simulink model "Longitudinal_Vehicle_Control"  (R2021a)
settings: Solver=VariableStepAuto  StartTime=0.0  StopTime=20  RelTol=1e-3
settings Model: Creator=AK  LastModifiedBy=AK

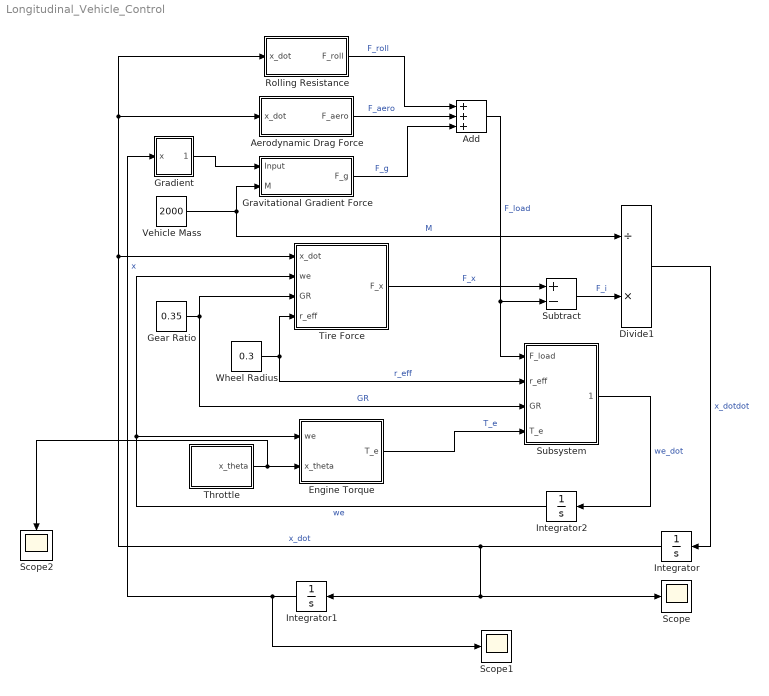
== system Longitudinal_Vehicle_Control ==
  Add : Sum  Inputs=+++
  Aerodynamic Drag Force : Subsystem
  Divide1 : Product  Inputs=/*
  Engine Torque : Subsystem
  Gear Ratio : Constant  Value=0.35
  Gradient : Subsystem
  Gravitational Gradient Force : Subsystem
  Integrator : Integrator  InitialCondition=5
  Integrator1 : Integrator
  Integrator2 : Integrator  InitialCondition=100
  Rolling Resistance : Subsystem
  Scope : Scope
  Scope1 : Scope
  Scope2 : Scope
  Subsystem : Subsystem
  Subtract : Sum  Inputs=+-
  Throttle : Subsystem
  Tire Force : Subsystem
  Vehicle Mass : Constant  Value=2000
  Wheel Radius : Constant  Value=0.3
  wires:
  Vehicle Mass/1 -> Divide1/1, Gravitational Gradient Force/2(M)  "M"
  Divide1/1 -> Integrator/1  "x_dotdot"
  Integrator/1 -> Scope/1, Integrator1/1, Tire Force/1(x_dot), Aerodynamic Drag Force/1(x_dot), Rolling Resistance/1(x_dot)  "x_dot"
  Add/1 -> Subtract/2, Subsystem/1(F_load)  "F_load"
  Gear Ratio/1 -> Subsystem/3(GR), Tire Force/3(GR)  "GR"
  Wheel Radius/1 -> Subsystem/2(r_eff), Tire Force/4(r_eff)  "r_eff"
  Integrator2/1 -> Tire Force/2(we), Engine Torque/1(we)  "we"
  Subtract/1 -> Divide1/2  "F_i"
  Aerodynamic Drag Force/1(F_aero) -> Add/2  "F_aero"
  Rolling Resistance/1(F_roll) -> Add/1  "F_roll"
  Gravitational Gradient Force/1(F_g) -> Add/3  "F_g"
  Tire Force/1(F_x) -> Subtract/1  "F_x"
  Engine Torque/1(T_e) -> Subsystem/4(T_e)  "T_e"
  Subsystem/1(we_dot) -> Integrator2/1  "we_dot"
  Integrator1/1 -> Scope1/1, Gradient/1(x)  "x"
  Gradient/1(alpha) -> Gravitational Gradient Force/1(Input)
  Throttle/1(x_theta) -> Scope2/1, Engine Torque/2(x_theta)

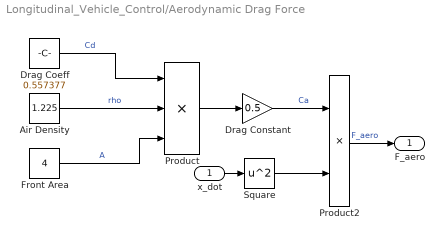
== system Longitudinal_Vehicle_Control/Aerodynamic Drag Force ==
  x_dot : Inport
  Air Density : Constant  Value=1.225
  Drag Coeff : Constant  Value=0.557377
  Drag Constant : Gain  Gain=0.5
  Front Area : Constant  Value=4
  Product : Product  Inputs=3
  Product2 : Product
  Square : Math  Operator=square  SaturateOnIntegerOverflow=on
  F_aero : Outport
  wires:
  Drag Constant/1 -> Product2/1  "Ca"
  Product/1 -> Drag Constant/1
  Air Density/1 -> Product/2  "rho"
  Drag Coeff/1 -> Product/1  "Cd"
  Square/1 -> Product2/2
  Product2/1 -> F_aero/1  "F_aero"
  Front Area/1 -> Product/3  "A"
  x_dot/1 -> Square/1

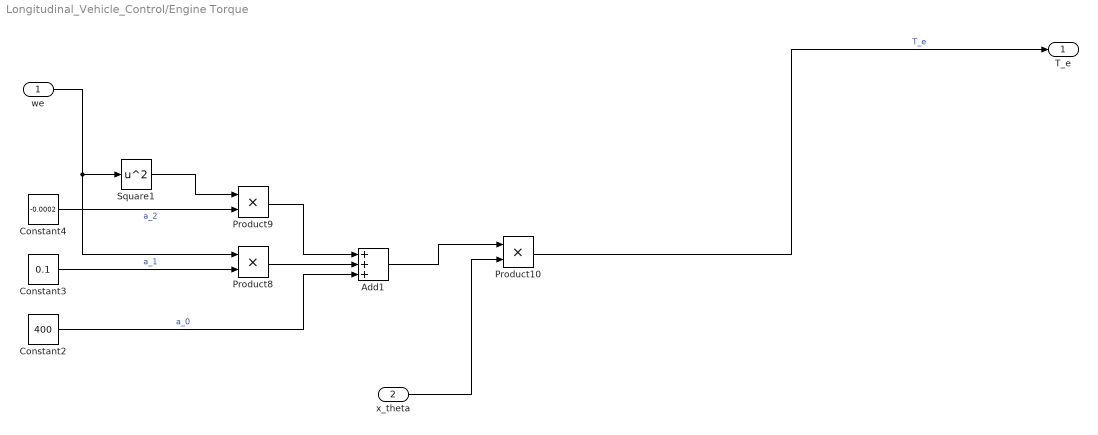
== system Longitudinal_Vehicle_Control/Engine Torque ==
  we : Inport
  x_theta : Inport  Port=2
  Add1 : Sum  Inputs=+++
  Constant2 : Constant  Value=400
  Constant3 : Constant  Value=0.1
  Constant4 : Constant  Value=-0.0002
  Product10 : Product
  Product8 : Product
  Product9 : Product
  Square1 : Math  Operator=square  SaturateOnIntegerOverflow=on
  T_e : Outport
  wires:
  Square1/1 -> Product9/1
  Add1/1 -> Product10/1
  Constant4/1 -> Product9/2  "a_2"
  we/1 -> Product8/1, Square1/1
  Product9/1 -> Add1/1
  Constant3/1 -> Product8/2  "a_1"
  Product8/1 -> Add1/2
  Constant2/1 -> Add1/3  "a_0"
  Product10/1 -> T_e/1  "T_e"
  x_theta/1 -> Product10/2

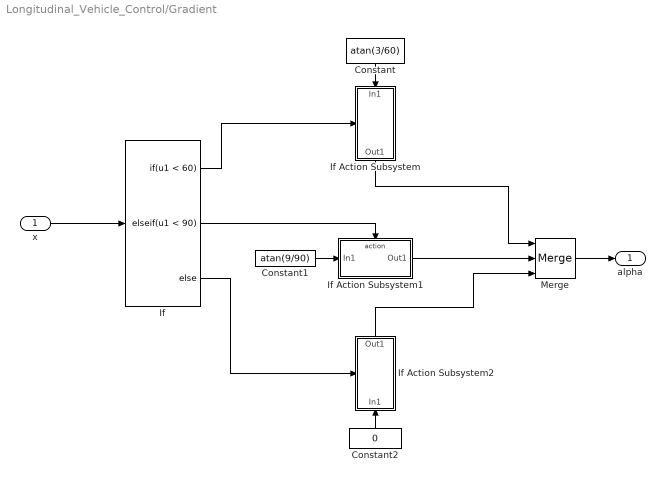
== system Longitudinal_Vehicle_Control/Gradient ==
  x : Inport
  Constant : Constant  Value=atan(3/60)
  Constant1 : Constant  Value=atan(9/90)
  Constant2 : Constant  Value=0
  If : If  IfExpression=u1 < 60  ElseIfExpressions=u1 < 90
  If Action Subsystem : Subsystem  TreatAsAtomicUnit=on
  If Action Subsystem1 : Subsystem  TreatAsAtomicUnit=on
  If Action Subsystem2 : Subsystem  TreatAsAtomicUnit=on
  Merge : Merge  Inputs=3
  alpha : Outport
  wires:
  x/1 -> If/1
  If/1 -> If Action Subsystem/Action
  Constant/1 -> If Action Subsystem/1(In1)
  Constant1/1 -> If Action Subsystem1/1(In1)
  If/2 -> If Action Subsystem1/Action
  Constant2/1 -> If Action Subsystem2/1(In1)
  If/3 -> If Action Subsystem2/Action
  If Action Subsystem/1(Out1) -> Merge/1
  If Action Subsystem1/1(Out1) -> Merge/2
  If Action Subsystem2/1(Out1) -> Merge/3
  Merge/1 -> alpha/1

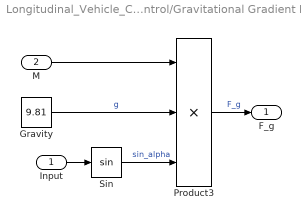
== system Longitudinal_Vehicle_Control/Gravitational Gradient Force ==
  Input : Inport
  M : Inport  Port=2
  Gravity : Constant  Value=9.81
  Product3 : Product  Inputs=3
  Sin : Trigonometry
  F_g : Outport
  wires:
  Sin/1 -> Product3/3  "sin_alpha"
  Gravity/1 -> Product3/2  "g"
  M/1 -> Product3/1
  Product3/1 -> F_g/1  "F_g"
  Input/1 -> Sin/1

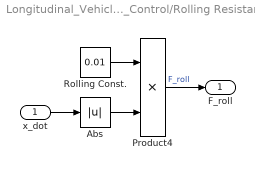
== system Longitudinal_Vehicle_Control/Rolling Resistance ==
  x_dot : Inport
  Abs : Abs
  Product4 : Product
  Rolling Const. : Constant  Value=0.01
  F_roll : Outport
  wires:
  Product4/1 -> F_roll/1  "F_roll"
  Rolling Const./1 -> Product4/1
  Abs/1 -> Product4/2
  x_dot/1 -> Abs/1

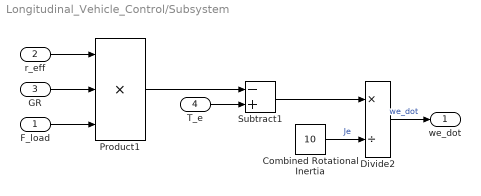
== system Longitudinal_Vehicle_Control/Subsystem ==
  F_load : Inport
  r_eff : Inport  Port=2
  GR : Inport  Port=3
  T_e : Inport  Port=4
  Combined Rotational Inertia : Constant  Value=10
  Divide2 : Product  Inputs=*/
  Product1 : Product  Inputs=3
  Subtract1 : Sum  Inputs=-+
  we_dot : Outport
  wires:
  r_eff/1 -> Product1/1
  Product1/1 -> Subtract1/1
  Combined Rotational Inertia/1 -> Divide2/2  "Je"
  Divide2/1 -> we_dot/1  "we_dot"
  GR/1 -> Product1/2
  T_e/1 -> Subtract1/2
  Subtract1/1 -> Divide2/1
  F_load/1 -> Product1/3

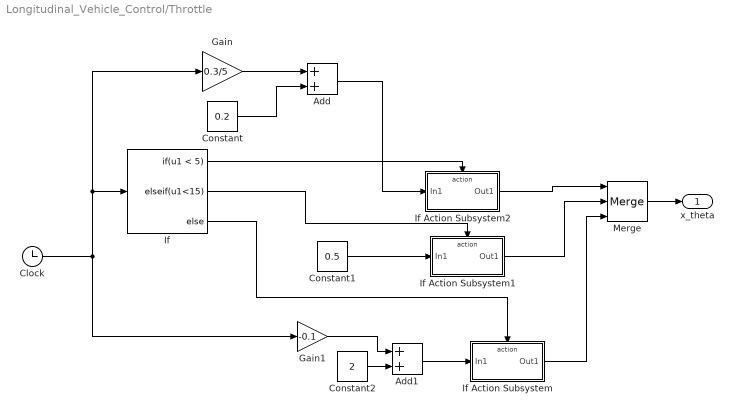
== system Longitudinal_Vehicle_Control/Throttle ==
  Add : Sum
  Add1 : Sum
  Clock : Clock
  Constant : Constant  Value=0.2
  Constant1 : Constant  Value=0.5
  Constant2 : Constant  Value=2
  Gain : Gain  Gain=0.3/5
  Gain1 : Gain  Gain=-0.1
  If : If  IfExpression=u1 < 5  ElseIfExpressions=u1<15
  If Action Subsystem : Subsystem  TreatAsAtomicUnit=on
  If Action Subsystem1 : Subsystem  TreatAsAtomicUnit=on
  If Action Subsystem2 : Subsystem  TreatAsAtomicUnit=on
  Merge : Merge  Inputs=3
  x_theta : Outport
  wires:
  Gain/1 -> Add/1
  Constant/1 -> Add/2
  Clock/1 -> If/1, Gain/1, Gain1/1
  Constant2/1 -> Add1/2
  Gain1/1 -> Add1/1
  Add1/1 -> If Action Subsystem/1(In1)
  If/3 -> If Action Subsystem/Action
  If Action Subsystem/1(Out1) -> Merge/3
  If/2 -> If Action Subsystem1/Action
  Constant1/1 -> If Action Subsystem1/1(In1)
  If Action Subsystem1/1(Out1) -> Merge/2
  If/1 -> If Action Subsystem2/Action
  Add/1 -> If Action Subsystem2/1(In1)
  If Action Subsystem2/1(Out1) -> Merge/1
  Merge/1 -> x_theta/1

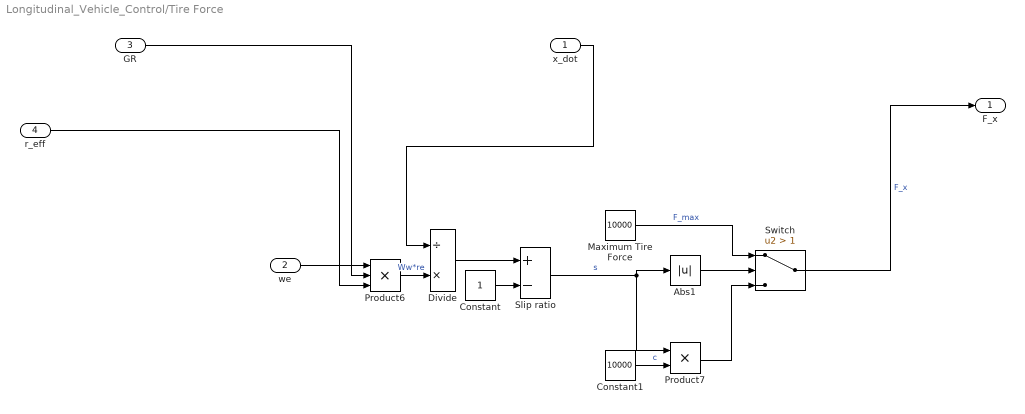
== system Longitudinal_Vehicle_Control/Tire Force ==
  x_dot : Inport
  we : Inport  Port=2
  GR : Inport  Port=3
  r_eff : Inport  Port=4
  Abs1 : Abs
  Constant : Constant
  Constant1 : Constant  Value=10000
  Divide : Product  Inputs=/*
  Maximum Tire Force : Constant  Value=10000
  Product6 : Product  Inputs=3
  Product7 : Product
  Slip ratio : Sum  Inputs=+-
  Switch : Switch  Criteria=u2 > Threshold  Threshold=1
  F_x : Outport
  wires:
  Constant/1 -> Slip ratio/2
  Divide/1 -> Slip ratio/1
  Product6/1 -> Divide/2  "Ww*re"
  Abs1/1 -> Switch/2
  Maximum Tire Force/1 -> Switch/1  "F_max"
  Product7/1 -> Switch/3
  Constant1/1 -> Product7/2  "c"
  Slip ratio/1 -> Abs1/1, Product7/1  "s"
  x_dot/1 -> Divide/1
  r_eff/1 -> Product6/3
  we/1 -> Product6/1
  Switch/1 -> F_x/1  "F_x"
  GR/1 -> Product6/2

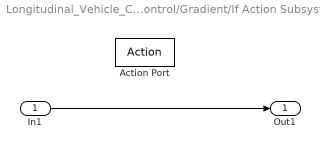
== system Longitudinal_Vehicle_Control/Gradient/If Action Subsystem ==
  In1 : Inport
  Action Port : ActionPort  ActionPortLabel=if(u1 < 60)
  Out1 : Outport
  wires:
  In1/1 -> Out1/1

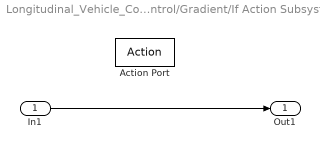
== system Longitudinal_Vehicle_Control/Gradient/If Action Subsystem1 ==
  In1 : Inport
  Action Port : ActionPort  ActionPortLabel=elseif(u1 < 90)
  Out1 : Outport
  wires:
  In1/1 -> Out1/1

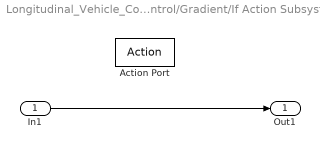
== system Longitudinal_Vehicle_Control/Gradient/If Action Subsystem2 ==
  In1 : Inport
  Action Port : ActionPort  ActionPortLabel=else
  Out1 : Outport
  wires:
  In1/1 -> Out1/1

== system Longitudinal_Vehicle_Control/Throttle/If Action Subsystem ==
  In1 : Inport
  Action Port : ActionPort  ActionPortLabel=else
  Out1 : Outport
  wires:
  In1/1 -> Out1/1

== system Longitudinal_Vehicle_Control/Throttle/If Action Subsystem1 ==
  In1 : Inport
  Action Port : ActionPort  ActionPortLabel=elseif(u1<15)
  Out1 : Outport
  wires:
  In1/1 -> Out1/1

== system Longitudinal_Vehicle_Control/Throttle/If Action Subsystem2 ==
  In1 : Inport
  Action Port : ActionPort  ActionPortLabel=if(u1 < 5)
  Out1 : Outport
  wires:
  In1/1 -> Out1/1
